simulink library "ddm"  (R2021b)
settings: Solver=VariableStepAuto  StartTime=0.0  StopTime=10.0  RelTol=1e-3
undefined symbols (not defined in the file or in its folder): ENUM_ADASACCSTA_ERROR, ENUM_ADASACCSTA_OFF, ENUM_ADASACCSTA_STANDBY, ENUM_ADASISASTA_OFF, ENUM_ALLOWMOV_ALLOWREADY, ENUM_APS, ENUM_BRKSTA_ERROR, ENUM_BRKSTA_OFF, ENUM_BRKSTA_ON, ENUM_CHGPREACTERRSTA_OBCPRE, ENUM_DCDCFAULTSTA_ANYFAULTLV1, ENUM_DCDCFAULTSTA_ANYFAULTLV2, ENUM_DRIVETRAIN_AWD, ENUM_DRIVETRAIN_FWD, ENUM_DRIVETRAIN_RWD, ENUM_DRSEATSTA_INVALID, ENUM_EDUDRTSTA_NORMAL, ENUM_EPBSTA_APPLIED, ENUM_EPBSTA_RELEASED, ENUM_HVBATTREADYPRE_READY, ENUM_MCUWARN_LV0, ENUM_MCUWARN_LV1, ENUM_MCUWARN_LV2, ENUM_MCUWARN_LV3, ENUM_MCUWARN_NOERROR, ENUM_OBCFAULTSTA_ANYFAULT, ENUM_PAS_R2F2, ENUM_PDFAULT_BATTPDFAIL, ENUM_PDFAULT_DCDCDISABLE, ENUM_PDFAULT_MCUDISABLE, ENUM_PDFAULT_MCUDISCHRG, ENUM_POWERSTA_OFF, ENUM_POWERSTA_ON, ENUM_POWERSTA_READY, ENUM_POWERSTA_STANDBY, ENUM_PRESSINDI_LOW, ENUM_PUFAULT_BATTUPFAIL, ENUM_PUFAULT_DCDCENABLEFAIL, ENUM_PUFAULT_PRECHRGCHKFAIL, ENUM_PUFAULT_SAFETYCHKFAIL, ENUM_PUSTATE_COMPLETED, ENUM_PWRSTASW_OFF, ENUM_PWRSTASW_OFFA, ENUM_PWRSTASW_OFFCHVCHRG, ENUM_PWRSTASW_OFFCLVCHRG, ENUM_PWRSTASW_ON, ENUM_PWRSTASW_ONHVCHRG, ENUM_PWRSTASW_READY, ENUM_PWRSTASW_STANDBY, ENUM_RANGESTA_12IN, ENUM_RANGESTA_12OUT, ENUM_SHIFTCOMMAND_D, ENUM_SHIFTCOMMAND_N, ENUM_SHIFTCOMMAND_P, ENUM_SHIFTCOMMAND_R, ENUM_ZONEMALFUNLV_1ST, ENUM_ZONEMALFUNLV_2ND, ENUM_ZONEMALFUNLV_3RD, ENUM_ZONEMALFUNLV_4TH, ENUM_ZONESPDCTRLMODE_ACC ... (+832)
libraries: hcu_lib x738, $bdroot x26, simulink x7
(part 11 of 25)

== system ddm/DDM/DDM/TQD/Shifter1_DDM ==
  note: Shifter1 Lost Comm (Shifter1NoCom)
  note: Shifter1 Rolling Count Error (Shifter1RCErr)
  note: Shifter1 Rolling Count Error (Shifter1CSErr)
  task_time_s : Inport
  VPMM_SysPwrSta_enum : Inport  Port=2
  No_CAN3_BUS_OFF : Inport  Port=3
  VDDM_Shifter1NoCom_flg : Inport  Port=4
  VDDM_Shifter1RCErr_flg : Inport  Port=5
  VDDM_Shifter1CSErr_flg : Inport  Port=6
  DTC_clear_request : Inport  Port=7
  Constant1 : Constant  Value=KDDM_Shifter1NoComCFSSW_flg
  Constant10 : Constant  Value=KDDM_Shifter1RCErrDFSSW_flg
  Constant{3,11,17,19,31,36} (6 alike) : Constant  Value=ENUM_PWRSTASW_OFF
  Constant12 : Constant  Value=FALSE
  Constant13 : Constant  Value=KDDM_Shifter1RCErrDTC_cnt
  Constant14 : Constant  Value=KDDM_Shifter1RCErrPassTO_s
  Constant15 : Constant  Value=KDDM_Shifter1NoComDTC_cnt
  Constant16 : Constant  Value=KDDM_Shifter1NoComDFSSW_flg
  Constant18 : Constant  Value=KDDM_Shifter1RCErrDetTO_s
  Constant2 : Constant  Value=FALSE
  Constant20 : Constant  Value=KDDM_Shifter1NoComDTC_cnt
  Constant21 : Constant  Value=KDDM_Shifter1NoComPassTO_s
  Constant22 : Constant  Value=KDDM_Shifter1NoComDetTO_s
  Constant23 : Constant  Value=ENUM_POWERSTA_OFF
  Constant24 : Constant  Value=ENUM_POWERSTA_STANDBY
  Constant25 : Constant  Value=KDDM_Shifter1RCErrDetSW_flg
  Constant26 : Constant  Value=KDDM_Shifter1RCErrPassSW_flg
  Constant27 : Constant  Value=KDDM_Shifter1RCErrPassTO_s
  Constant28 : Constant  Value=KDDM_Shifter1CSErrCFSSW_flg
  Constant29 : Constant  Value=KDDM_Shifter1CSErrDTC_cnt
  Constant30 : Constant  Value=KDDM_Shifter1CSErrDFSSW_flg
  Constant32 : Constant  Value=FALSE
  Constant33 : Constant  Value=KDDM_Shifter1CSErrDTC_cnt
  Constant34 : Constant  Value=KDDM_Shifter1CSErrPassTO_s
  Constant35 : Constant  Value=KDDM_Shifter1CSErrDetTO_s
  Constant37 : Constant  Value=ENUM_POWERSTA_OFF
  Constant38 : Constant  Value=ENUM_POWERSTA_STANDBY
  Constant39 : Constant  Value=KDDM_Shifter1CSErrDetSW_flg
  Constant4 : Constant  Value=ENUM_POWERSTA_OFF
  Constant40 : Constant  Value=KDDM_Shifter1CSErrPassSW_flg
  Constant41 : Constant  Value=KDDM_Shifter1CSErrPassTO_s
  Constant5 : Constant  Value=ENUM_POWERSTA_STANDBY
  Constant6 : Constant  Value=KDDM_Shifter1NoComDetSW_flg
  Constant7 : Constant  Value=KDDM_Shifter1NoComPassSW_flg
  Constant70 : Constant  Value=KDDM_Shifter1NoComPassTO_s
  Constant8 : Constant  Value=KDDM_Shifter1RCErrCFSSW_flg
  Constant9 : Constant  Value=KDDM_Shifter1RCErrDTC_cnt
  DTC_Couter1 : hcu_lib/Basic_Blocks/DTC_Couter
  DTC_Couter2 : hcu_lib/Basic_Blocks/DTC_Couter
  DTC_Couter3 : hcu_lib/Basic_Blocks/DTC_Couter
  DTC_Info : hcu_lib/Basic_Blocks/DTC_Info
  DTC_Info1 : hcu_lib/Basic_Blocks/DTC_Info
  DTC_Info2 : hcu_lib/Basic_Blocks/DTC_Info
  Data Type Conversion1 : DataTypeConversion  OutDataTypeStr=uint8
  Data Type Conversion2 : DataTypeConversion  OutDataTypeStr=uint8
  Data Type Conversion3 : DataTypeConversion  OutDataTypeStr=uint8
  Equal{1,3,9..12} (6 alike) : RelationalOperator  Operator===  OutDataTypeStr=boolean  RndMeth=Simplest
  Equal{2,4..6,13..14} (6 alike) : RelationalOperator  Operator=~=  OutDataTypeStr=boolean  RndMeth=Simplest
  Equal15 : RelationalOperator  OutDataTypeStr=boolean  RndMeth=Simplest
  Equal7 : RelationalOperator  OutDataTypeStr=boolean  RndMeth=Simplest
  Equal8 : RelationalOperator  OutDataTypeStr=boolean  RndMeth=Simplest
  Logical Operator{1,3,5,11,23,25,27,37,77} (9 alike) : Logic  Operator=OR  AllPortsSameDT=off  OutDataTypeStr=boolean
  Logical Operator10 : Logic  Inputs=3  AllPortsSameDT=off  OutDataTypeStr=boolean
  Logical Operator{6,9,12,14,20,24,28,30,34,38} (10 alike) : Logic  Operator=NOT  AllPortsSameDT=off  OutDataTypeStr=boolean
  Logical Operator{2,8,13,15..19,21,29,31..33,35,55} (15 alike) : Logic  AllPortsSameDT=off  OutDataTypeStr=boolean
  Logical Operator{4,22,26,36} (4 alike) : Logic  Inputs=4  AllPortsSameDT=off  OutDataTypeStr=boolean
  Logical Operator7 : Logic  Inputs=3  AllPortsSameDT=off  OutDataTypeStr=boolean
  Relay1 : Relay  OnSwitchValue=ONE_INT  OffSwitchValue=ZERO_INT
  Relay2 : Relay  OnSwitchValue=ONE_INT  OffSwitchValue=ZERO_INT
  Relay3 : Relay  OnSwitchValue=ONE_INT  OffSwitchValue=ZERO_INT
  SR_Latch{1..8,12} (9 alike) : hcu_lib/Basic_Blocks/SR_Latch
  Switch1 : Switch  Criteria=u2 ~= 0
  Switch2 : Switch  Criteria=u2 ~= 0
  Switch6 : Switch  Criteria=u2 ~= 0
  Test Detection Criteria1 : hcu_lib/Basic_Blocks/Test Detection Criteria
  Test Detection Criteria2 : hcu_lib/Basic_Blocks/Test Detection Criteria
  Test Detection Criteria3 : hcu_lib/Basic_Blocks/Test Detection Criteria
  Timer1 : hcu_lib/Basic_Blocks/Timer
  Timer2 : hcu_lib/Basic_Blocks/Timer
  Timer3 : hcu_lib/Basic_Blocks/Timer
  Unit Delay1 : UnitDelay  SampleTime=-1  HasFrameUpgradeWarning=on
  Unit Delay2 : UnitDelay  SampleTime=-1  HasFrameUpgradeWarning=on
  Unit Delay3 : UnitDelay  SampleTime=-1  HasFrameUpgradeWarning=on
  VDDM_Shifter1NoComDTC_raw32 : Outport
  VDDM_Shifter1RCErrDTC_raw32 : Outport  Port=2
  VDDM_Shifter1CSErrDTC_raw32 : Outport  Port=3
  wires:
  Logical Operator77/1 -> SR_Latch2/2
  [DTC_clear_request] -> Logical Operator1/2
  SR_Latch2/1 -> Logical Operator55/2
  Logical Operator14/1 -> Timer2/2
  [VDDM_Shifter1NoComCFSRls_flg] -> SR_Latch1/2
  Logical Operator13/1 -> Logical Operator1/1
  Relay1/1 -> SR_Latch2/1
  Constant22/1 -> Test Detection Criteria1/4
  Logical Operator16/1 -> DTC_Couter1/2
  Logical Operator7/1 -> Logical Operator14/1, Timer2/1
  Timer2/1 -> Equal7/1
  Equal10/1 -> Logical Operator13/1
  SR_Latch12/1 -> [VDDM_Shifter1NoComPass_flg]
  DTC_Couter1/2 -> Data Type Conversion2/1
  Constant4/1 -> Equal10/2
  [VDDM_Shifter1NoComDet_flg] -> Logical Operator15/1
  Constant6/1 -> Logical Operator15/2
  Test Detection Criteria1/1 -> [VDDM_Shifter1NoComDet_flg]  "VDDM_Shifter1NoComDet_flg"
  Logical Operator15/1 -> DTC_Couter1/1
  [VDDM_Shifter1NoComCFSRls_flg] -> Logical Operator11/2
  [VDDM_Shifter1NoComDFSRls_flg] -> Logical Operator77/1
  [VDDM_Shifter1NoComPass_flg] -> Logical Operator11/1
  [VDDM_Shifter1NoComDTC_cnt] -> Relay1/1
  Constant20/1 -> Test Detection Criteria1/3
  [VDDM_Shifter1NoComCFS_flg] -> Logical Operator77/2
  [VPMM_SysPwrSta_enum] -> Equal11/1
  Equal7/1 -> SR_Latch12/1
  Equal11/1 -> Logical Operator13/2
  Unit Delay2/1 -> Equal10/1
  Logical Operator11/1 -> Logical Operator16/1
  Constant16/1 -> Logical Operator55/1
  Data Type Conversion2/1 -> [VDDM_Shifter1NoComDTC_cnt]  "VDDM_Shifter1NoComDTC_cnt"
  Logical Operator55/1 -> [VDDM_Shifter1NoComDFS_flg]
  Constant15/1 -> DTC_Couter1/3
  Constant5/1 -> Equal11/2
  Constant7/1 -> Logical Operator16/2
  Logical Operator1/1 -> [VDDM_Shifter1NoComCFSRls_flg]
  Constant70/1 -> Timer2/4
  DTC_Couter1/1 -> SR_Latch1/1
  [VPMM_SysPwrSta_enum] -> Unit Delay2/1
  [task_time_s] -> Test Detection Criteria1/2
  Constant21/1 -> Equal7/2
  [task_time_s] -> Timer2/3
  [No_CAN3_BUS_OFF] -> Logical Operator10/2
  Equal6/1 -> Logical Operator10/1
  Constant17/1 -> Equal6/2
  [VDDM_Shifter1NoCom_flg] -> Logical Operator10/3
  [VPMM_SysPwrSta_enum] -> Equal6/1
  [VDDM_Shifter1NoCom_flg] -> Logical Operator9/1
  Equal2/1 -> Logical Operator7/1
  Logical Operator9/1 -> Logical Operator7/3
  Constant3/1 -> Equal2/2
  [No_CAN3_BUS_OFF] -> Logical Operator7/2
  [VPMM_SysPwrSta_enum] -> Equal2/1
  VDDM_Shifter1NoCom_flg/1 -> [VDDM_Shifter1NoCom_flg]
  VPMM_SysPwrSta_enum/1 -> [VPMM_SysPwrSta_enum]
  [VDDM_Shifter1NoComCFS_flg] -> DTC_Info/3
  DTC_Info/1 -> VDDM_Shifter1NoComDTC_raw32/1  "VDDM_Shifter1NoComDTC_raw32"
  [VDDM_Shifter1NoComPass_flg] -> DTC_Info/2
  task_time_s/1 -> [task_time_s]
  DTC_clear_request/1 -> [DTC_clear_request]
  [VDDM_Shifter1NoComDet_flg] -> DTC_Info/1
  No_CAN3_BUS_OFF/1 -> [No_CAN3_BUS_OFF]
  Constant1/1 -> Logical Operator2/2
  Logical Operator2/1 -> [VDDM_Shifter1NoComCFS_flg]
  SR_Latch1/1 -> Logical Operator2/1
  [DTC_clear_request] -> DTC_Info/4
  [DTC_clear_request] -> Switch6/2
  Switch6/1 -> Test Detection Criteria1/1
  Logical Operator10/1 -> [VDDM_Shifter1NoComRst_flg], Switch6/3
  Constant2/1 -> Switch6/1
  Logical Operator20/1 -> Logical Operator4/4
  [DTC_clear_request] -> Logical Operator3/2
  Constant26/1 -> Logical Operator18/2
  Logical Operator12/1 -> Timer1/2
  SR_Latch5/1 -> Logical Operator21/2
  [VPMM_SysPwrSta_enum] -> Equal4/1
  [VDDM_Shifter1RCErrPass_flg] -> Logical Operator5/1
  Logical Operator8/1 -> Logical Operator3/1
  Logical Operator19/1 -> [VDDM_Shifter1RCErrCFS_flg]
  Constant13/1 -> Test Detection Criteria2/3
  Equal1/1 -> Logical Operator8/1
  Constant25/1 -> Logical Operator17/2
  Logical Operator5/1 -> Logical Operator18/1
  SR_Latch4/1 -> [VDDM_Shifter1RCErrPass_flg]
  Logical Operator17/1 -> DTC_Couter2/1
  [VDDM_Shifter1RCErrCFS_flg] -> Logical Operator23/2
  DTC_Couter2/2 -> Data Type Conversion1/1
  Equal5/1 -> Logical Operator4/1
  Logical Operator22/1 -> Timer1/1, Logical Operator12/1
  Unit Delay1/1 -> Equal1/1
  [VDDM_Shifter1NoComCFS_flg] -> Logical Operator20/1
  Constant24/1 -> Equal3/2
  Logical Operator21/1 -> [VDDM_Shifter1RCErrDFS_flg]
  Constant14/1 -> Equal8/2
  [VDDM_Shifter1RCErr_flg] -> Logical Operator24/1
  Logical Operator3/1 -> [VDDM_Shifter1RCErrCFSRls_flg]
  Constant19/1 -> Equal4/2
  Equal8/1 -> SR_Latch4/1
  [VDDM_Shifter1RCErrCFSRls_flg] -> SR_Latch3/2
  Constant11/1 -> Equal5/2
  Constant18/1 -> Test Detection Criteria2/4
  [VDDM_Shifter1RCErrPass_flg] -> DTC_Info1/2
  [No_CAN3_BUS_OFF] -> Logical Operator22/2
  Equal4/1 -> Logical Operator22/1
  Constant23/1 -> Equal1/2
  Logical Operator18/1 -> DTC_Couter2/2
  Data Type Conversion1/1 -> [VDDM_Shifter1RCErrDTC_cnt]  "VDDM_Shifter1RCErrDTC_cnt"
  DTC_Info1/1 -> VDDM_Shifter1RCErrDTC_raw32/1  "VDDM_Shifter1RCErrDTC_raw32"
  Constant10/1 -> Logical Operator21/1
  Logical Operator23/1 -> SR_Latch5/2
  [VPMM_SysPwrSta_enum] -> Equal3/1
  [VPMM_SysPwrSta_enum] -> Equal5/1
  [No_CAN3_BUS_OFF] -> Logical Operator4/2
  [VDDM_Shifter1RCErrDet_flg] -> DTC_Info1/1
  Relay2/1 -> SR_Latch5/1
  [VDDM_Shifter1RCErrDet_flg] -> Logical Operator17/1
  [task_time_s] -> Timer1/3
  [task_time_s] -> Test Detection Criteria2/2
  Constant27/1 -> Timer1/4
  Timer1/1 -> Equal8/1
  SR_Latch3/1 -> Logical Operator19/1
  [DTC_clear_request] -> Switch1/2
  Constant12/1 -> Switch1/1
  Equal3/1 -> Logical Operator8/2
  [VDDM_Shifter1RCErrDTC_cnt] -> Relay2/1
  [VDDM_Shifter1RCErrCFS_flg] -> DTC_Info1/3
  [VPMM_SysPwrSta_enum] -> Unit Delay1/1
  Constant9/1 -> DTC_Couter2/3
  Logical Operator4/1 -> [VDDM_Shifter1RCErrRst_flg], Switch1/3
  [VDDM_Shifter1RCErrDFSRls_flg] -> Logical Operator23/1
  [VDDM_Shifter1RCErrCFSRls_flg] -> Logical Operator5/2
  Logical Operator24/1 -> Logical Operator22/3
  DTC_Couter2/1 -> SR_Latch3/1
  [DTC_clear_request] -> DTC_Info1/4
  Constant8/1 -> Logical Operator19/2
  [VDDM_Shifter1RCErr_flg] -> Logical Operator4/3
  Test Detection Criteria2/1 -> [VDDM_Shifter1RCErrDet_flg]  "VDDM_Shifter1RCErrDet_flg"
  Logical Operator34/1 -> Logical Operator26/4
  [DTC_clear_request] -> Logical Operator25/2
  Constant40/1 -> Logical Operator32/2
  Logical Operator30/1 -> Timer3/2
  SR_Latch8/1 -> Logical Operator35/2
  [VPMM_SysPwrSta_enum] -> Equal13/1
  [VDDM_Shifter1CSErrPass_flg] -> Logical Operator27/1
  Logical Operator29/1 -> Logical Operator25/1
  Logical Operator33/1 -> [VDDM_Shifter1CSErrCFS_flg]
  Constant33/1 -> Test Detection Criteria3/3
  Equal9/1 -> Logical Operator29/1
  Constant39/1 -> Logical Operator31/2
  Logical Operator27/1 -> Logical Operator32/1
  SR_Latch7/1 -> [VDDM_Shifter1CSErrPass_flg]
  Logical Operator31/1 -> DTC_Couter3/1
  [VDDM_Shifter1CSErrCFS_flg] -> Logical Operator37/2
  DTC_Couter3/2 -> Data Type Conversion3/1
  Equal14/1 -> Logical Operator26/1
  Logical Operator36/1 -> Timer3/1, Logical Operator30/1
  Unit Delay3/1 -> Equal9/1
  [VDDM_Shifter1NoComCFS_flg] -> Logical Operator34/1
  Constant38/1 -> Equal12/2
  Logical Operator35/1 -> [VDDM_Shifter1CSErrDFS_flg]
  Constant34/1 -> Equal15/2
  [VDDM_Shifter1CSErr_flg] -> Logical Operator38/1
  Logical Operator25/1 -> [VDDM_Shifter1CSErrCFSRls_flg]
  Constant36/1 -> Equal13/2
  Equal15/1 -> SR_Latch7/1
  [VDDM_Shifter1CSErrCFSRls_flg] -> SR_Latch6/2
  Constant31/1 -> Equal14/2
  Constant35/1 -> Test Detection Criteria3/4
  [VDDM_Shifter1CSErrPass_flg] -> DTC_Info2/2
  [No_CAN3_BUS_OFF] -> Logical Operator36/2
  Equal13/1 -> Logical Operator36/1
  Constant37/1 -> Equal9/2
  Logical Operator32/1 -> DTC_Couter3/2
  Data Type Conversion3/1 -> [VDDM_Shifter1CSErrDTC_cnt]  "VDDM_Shifter1CSErrDTC_cnt"
  DTC_Info2/1 -> VDDM_Shifter1CSErrDTC_raw32/1  "VDDM_Shifter1CSErrDTC_raw32"
  Constant30/1 -> Logical Operator35/1
  Logical Operator37/1 -> SR_Latch8/2
  [VPMM_SysPwrSta_enum] -> Equal12/1
  [VPMM_SysPwrSta_enum] -> Equal14/1
  [No_CAN3_BUS_OFF] -> Logical Operator26/2
  [VDDM_Shifter1CSErrDet_flg] -> DTC_Info2/1
  Relay3/1 -> SR_Latch8/1
  [VDDM_Shifter1CSErrDet_flg] -> Logical Operator31/1
  [task_time_s] -> Timer3/3
  [task_time_s] -> Test Detection Criteria3/2
  Constant41/1 -> Timer3/4
  Timer3/1 -> Equal15/1
  SR_Latch6/1 -> Logical Operator33/1
  [DTC_clear_request] -> Switch2/2
  Constant32/1 -> Switch2/1
  Equal12/1 -> Logical Operator29/2
  [VDDM_Shifter1CSErrDTC_cnt] -> Relay3/1
  [VDDM_Shifter1CSErrCFS_flg] -> DTC_Info2/3
  [VPMM_SysPwrSta_enum] -> Unit Delay3/1
  Constant29/1 -> DTC_Couter3/3
  Logical Operator26/1 -> [VDDM_Shifter1CSErrRst_flg], Switch2/3
  [VDDM_Shifter1CSErrDFSRls_flg] -> Logical Operator37/1
  [VDDM_Shifter1CSErrCFSRls_flg] -> Logical Operator27/2
  Logical Operator38/1 -> Logical Operator36/3
  DTC_Couter3/1 -> SR_Latch6/1
  [DTC_clear_request] -> DTC_Info2/4
  Constant28/1 -> Logical Operator33/2
  [VDDM_Shifter1CSErr_flg] -> Logical Operator26/3
  Test Detection Criteria3/1 -> [VDDM_Shifter1CSErrDet_flg]  "VDDM_Shifter1CSErrDet_flg"
  [VDDM_Shifter1NoComRst_flg] -> SR_Latch12/2
  Switch1/1 -> Test Detection Criteria2/1
  [VDDM_Shifter1RCErrRst_flg] -> SR_Latch4/2
  [VDDM_Shifter1CSErrRst_flg] -> SR_Latch7/2
  Switch2/1 -> Test Detection Criteria3/1
  VDDM_Shifter1RCErr_flg/1 -> [VDDM_Shifter1RCErr_flg]
  VDDM_Shifter1CSErr_flg/1 -> [VDDM_Shifter1CSErr_flg]
  [VDDM_Shifter1NoComCFS_flg] -> Logical Operator6/1
  Logical Operator6/1 -> Logical Operator22/4
  [VDDM_Shifter1NoComCFS_flg] -> Logical Operator28/1
  Logical Operator28/1 -> Logical Operator36/4

== system ddm/DDM/DDM/VMC_DDM/ACC Acceleration Command Error ==
  task_time_s : Inport
  VDDM_FCM2NoComCFS_flg : Inport  Port=2
  VDDM_FCM2RCErrCFS_flg : Inport  Port=3
  VDDM_FCM2CSErrCFS_flg : Inport  Port=4
  VVMC_ADASActive_flg : Inport  Port=5
  No_CAN_BUS_OFF : Inport  Port=6
  VPMM_PowerSta_enum : Inport  Port=7
  VINP_ACCRequireAccel_mps2 : Inport  Port=8
  VINP_ADASACCSta_enum : Inport  Port=9
  DTC_clear_request : Inport  Port=10
  "ACC Acceleration Command Error " : Subsystem
  From5 : From  Commented=on  GotoTag=VDDM_ACCAccelCmdErrDFS_flg
  Terminator : Terminator
  VDDM_ACCAccelCmdErrCFS_flg : Outport
  VDDM_ACCAccelCmdErrDetDTC_raw32 : Outport  Port=2
  wires:
  VDDM_FCM2CSErrCFS_flg/1 -> [VDDM_FCM2CSErrCFS_flg]
  VDDM_FCM2RCErrCFS_flg/1 -> [VDDM_FCM2RCErrCFS_flg]
  [VDDM_ACCAccelCmdErrCFS_flg] -> VDDM_ACCAccelCmdErrCFS_flg/1
  From5/1 -> Terminator/1
  "ACC Acceleration Command Error "/1(VDDM_ACCAccelCmdErrCFS_flg) -> [VDDM_ACCAccelCmdErrCFS_flg]
  DTC_clear_request/1 -> [DTC_clear_request]
  VPMM_PowerSta_enum/1 -> [VPMM_PowerSta_enum]
  No_CAN_BUS_OFF/1 -> [No_CAN_BUS_OFF]
  VDDM_FCM2NoComCFS_flg/1 -> [VDDM_FCM2NoComCFS_flg]
  VINP_ACCRequireAccel_mps2/1 -> [VINP_ACCRequireAccel_mps2]
  [VDDM_FCM2NoComCFS_flg] -> "ACC Acceleration Command Error "/2(VDDM_FCM2NoComCFS_flg)
  [VDDM_FCM2RCErrCFS_flg] -> "ACC Acceleration Command Error "/3(VDDM_FCM2RCErrCFS_flg)
  [VDDM_FCM2CSErrCFS_flg] -> "ACC Acceleration Command Error "/4(VDDM_FCM2CSErrCFS_flg)
  [No_CAN_BUS_OFF] -> "ACC Acceleration Command Error "/6(No_CAN_BUS_OFF)
  [VPMM_PowerSta_enum] -> "ACC Acceleration Command Error "/7(VPMM_PowerSta_enum)
  [VINP_ACCRequireAccel_mps2] -> "ACC Acceleration Command Error "/8(VINP_ACCRequireAccel_mps2)
  [DTC_clear_request] -> "ACC Acceleration Command Error "/10(DTC_clear_request)
  task_time_s/1 -> [task_time_s]  "task_time_s"
  [task_time_s] -> "ACC Acceleration Command Error "/1(task_time_s)
  VVMC_ADASActive_flg/1 -> [VVMC_ADASActive_flg]
  [VVMC_ADASActive_flg] -> "ACC Acceleration Command Error "/5(VVMC_ADASActive_flg)
  [VINP_ADASACCSta_enum] -> "ACC Acceleration Command Error "/9(VINP_ADASACCSta_enum)
  VINP_ADASACCSta_enum/1 -> [VINP_ADASACCSta_enum]
  "ACC Acceleration Command Error "/2(VDDM_ACCAccelCmdErrDetDTC_raw32) -> [VDDM_ACCAccelCmdErrDetDTC_raw32]
  [VDDM_ACCAccelCmdErrDetDTC_raw32] -> VDDM_ACCAccelCmdErrDetDTC_raw32/1

== system ddm/DDM/DDM/VMC_DDM/ACC Malfunction  ==
  task_time_s : Inport
  VDDM_FCMACCSigErrCFS_flg : Inport  Port=2
  VDDM_ACCAccelCmdErrCFS_flg : Inport  Port=3
  VDDM_BMSSigErrCFS_flg : Inport  Port=4
  VDDM_FrMCUSigErrCFS_flg : Inport  Port=5
  VDDM_RrMCUSigErrCFS_flg : Inport  Port=6
  VDDM_CCUSigErrCFS_flg : Inport  Port=7
  VDDM_FCM2NoComCFS_flg : Inport  Port=8
  VDDM_FCM2RCErrCFS_flg : Inport  Port=9
  VDDM_FCM2CSErrCFS_flg : Inport  Port=10
  VDDM_FCM4NoComCFS_flg : Inport  Port=11
  VDDM_FCM4CSErrCFS_flg : Inport  Port=12
  VDDM_ZoneSCPNoComCFS_flg : Inport  Port=13
  VDDM_MCUR1NoComCFS_flg : Inport  Port=14
  VDDM_MCUR1RCErrCFS_flg : Inport  Port=15
  VDDM_MCUR1CSErrCFS_flg : Inport  Port=16
  VDDM_MCUF1NoComCFS_flg : Inport  Port=17
  VDDM_MCUF1RCErrCFS_flg : Inport  Port=18
  VDDM_MCUF1CSErrCFS_flg : Inport  Port=19
  VDDM_ESC7NoComCFS_flg : Inport  Port=20
  VDDM_ESC7RCErrCFS_flg : Inport  Port=21
  VDDM_ESC7CSErrCFS_flg : Inport  Port=22
  VDDM_ESC1NoComCFS_flg : Inport  Port=23
  VDDM_ESC1RCErrCFS_flg : Inport  Port=24
  VDDM_ESC1CSErrCFS_flg : Inport  Port=25
  VDDM_ESC5NoComCFS_flg : Inport  Port=26
  VDDM_ESC5RCErrCFS_flg : Inport  Port=27
  VDDM_ESC5CSErrCFS_flg : Inport  Port=28
  No_CAN1_BUS_OFF : Inport  Port=29
  No_CAN3_BUS_OFF : Inport  Port=30
  No_CAN4_BUS_OFF : Inport  Port=31
  VPMM_PowerSta_enum : Inport  Port=32
  VINP_ZoneSpdCtrlMode_enum : Inport  Port=33
  DTC_clear_request : Inport  Port=34
  "ACC Malfunction " : Subsystem
  From5 : From  Commented=on  GotoTag=VDDM_ACCMalfuncDFS_flg
  Terminator : Terminator
  VDDM_ACCMalfuncCFS_flg : Outport
  VDDM_ACCMalfuncDetDTC_raw32 : Outport  Port=2
  wires:
  VDDM_BMSSigErrCFS_flg/1 -> [VDDM_BMSSigErrCFS_flg]
  VDDM_ACCAccelCmdErrCFS_flg/1 -> [VDDM_ACCAccelCmdErrCFS_flg]
  [VDDM_ACCMalfuncCFS_flg] -> VDDM_ACCMalfuncCFS_flg/1
  From5/1 -> Terminator/1
  "ACC Malfunction "/1(VDDM_ACCMalfuncCFS_flg) -> [VDDM_ACCMalfuncCFS_flg]
  VPMM_PowerSta_enum/1 -> [VPMM_PowerSta_enum]
  No_CAN1_BUS_OFF/1 -> [No_CAN1_BUS_OFF]
  VDDM_FCMACCSigErrCFS_flg/1 -> [VDDM_FCMACCSigErrCFS_flg]
  VINP_ZoneSpdCtrlMode_enum/1 -> [VINP_ZoneSpdCtrlMode_enum]
  task_time_s/1 -> [task_time_s]  "task_time_s"
  VDDM_FrMCUSigErrCFS_flg/1 -> [VDDM_FrMCUSigErrCFS_flg]
  VDDM_RrMCUSigErrCFS_flg/1 -> [VDDM_RrMCUSigErrCFS_flg]
  VDDM_CCUSigErrCFS_flg/1 -> [VDDM_CCUSigErrCFS_flg]
  VDDM_ZoneSCPNoComCFS_flg/1 -> [VDDM_ZoneSCPNoComCFS_flg]
  VDDM_FCM4CSErrCFS_flg/1 -> [VDDM_FCM4CSErrCFS_flg]
  VDDM_FCM4NoComCFS_flg/1 -> [VDDM_FCM4NoComCFS_flg]
  VDDM_FCM2NoComCFS_flg/1 -> [VDDM_FCM2NoComCFS_flg]
  VDDM_FCM2RCErrCFS_flg/1 -> [VDDM_FCM2RCErrCFS_flg]
  VDDM_FCM2CSErrCFS_flg/1 -> [VDDM_FCM2CSErrCFS_flg]
  VDDM_ESC7CSErrCFS_flg/1 -> [VDDM_ESC7CSErrCFS_flg]
  VDDM_ESC7RCErrCFS_flg/1 -> [VDDM_ESC7RCErrCFS_flg]
  VDDM_ESC7NoComCFS_flg/1 -> [VDDM_ESC7NoComCFS_flg]
  VDDM_ESC1NoComCFS_flg/1 -> [VDDM_ESC1NoComCFS_flg]
  VDDM_ESC1RCErrCFS_flg/1 -> [VDDM_ESC1RCErrCFS_flg]
  VDDM_ESC1CSErrCFS_flg/1 -> [VDDM_ESC1CSErrCFS_flg]
  VDDM_MCUF1CSErrCFS_flg/1 -> [VDDM_MCUF1CSErrCFS_flg]
  VDDM_MCUF1RCErrCFS_flg/1 -> [VDDM_MCUF1RCErrCFS_flg]
  VDDM_MCUF1NoComCFS_flg/1 -> [VDDM_MCUF1NoComCFS_flg]
  VDDM_MCUR1NoComCFS_flg/1 -> [VDDM_MCUR1NoComCFS_flg]
  VDDM_MCUR1RCErrCFS_flg/1 -> [VDDM_MCUR1RCErrCFS_flg]
  VDDM_MCUR1CSErrCFS_flg/1 -> [VDDM_MCUR1CSErrCFS_flg]
  VDDM_ESC5CSErrCFS_flg/1 -> [VDDM_ESC5CSErrCFS_flg]
  VDDM_ESC5RCErrCFS_flg/1 -> [VDDM_ESC5RCErrCFS_flg]
  VDDM_ESC5NoComCFS_flg/1 -> [VDDM_ESC5NoComCFS_flg]
  No_CAN3_BUS_OFF/1 -> [No_CAN3_BUS_OFF]
  No_CAN4_BUS_OFF/1 -> [No_CAN4_BUS_OFF]
  DTC_clear_request/1 -> [DTC_clear_request]
  [No_CAN3_BUS_OFF] -> "ACC Malfunction "/30(No_CAN3_BUS_OFF)
  [VDDM_MCUR1CSErrCFS_flg] -> "ACC Malfunction "/16(VDDM_MCUR1CSErrCFS_flg)
  [VDDM_RrMCUSigErrCFS_flg] -> "ACC Malfunction "/6(VDDM_RrMCUSigErrCFS_flg)
  [VDDM_BMSSigErrCFS_flg] -> "ACC Malfunction "/4(VDDM_BMSSigErrCFS_flg)
  [VDDM_MCUF1NoComCFS_flg] -> "ACC Malfunction "/17(VDDM_MCUF1NoComCFS_flg)
  [No_CAN4_BUS_OFF] -> "ACC Malfunction "/31(No_CAN4_BUS_OFF)
  [VDDM_FrMCUSigErrCFS_flg] -> "ACC Malfunction "/5(VDDM_FrMCUSigErrCFS_flg)
  [DTC_clear_request] -> "ACC Malfunction "/34(DTC_clear_request)
  [VDDM_ACCAccelCmdErrCFS_flg] -> "ACC Malfunction "/3(VDDM_ACCAccelCmdErrCFS_flg)
  [VDDM_MCUF1RCErrCFS_flg] -> "ACC Malfunction "/18(VDDM_MCUF1RCErrCFS_flg)
  [VDDM_ESC7CSErrCFS_flg] -> "ACC Malfunction "/22(VDDM_ESC7CSErrCFS_flg)
  [VDDM_FCM4CSErrCFS_flg] -> "ACC Malfunction "/12(VDDM_FCM4CSErrCFS_flg)
  [VDDM_ESC1RCErrCFS_flg] -> "ACC Malfunction "/24(VDDM_ESC1RCErrCFS_flg)
  [VDDM_ESC7RCErrCFS_flg] -> "ACC Malfunction "/21(VDDM_ESC7RCErrCFS_flg)
  [VDDM_ESC7NoComCFS_flg] -> "ACC Malfunction "/20(VDDM_ESC7NoComCFS_flg)
  [VDDM_ESC5CSErrCFS_flg] -> "ACC Malfunction "/28(VDDM_ESC5CSErrCFS_flg)
  [VDDM_ESC5RCErrCFS_flg] -> "ACC Malfunction "/27(VDDM_ESC5RCErrCFS_flg)
  [VDDM_ESC1NoComCFS_flg] -> "ACC Malfunction "/23(VDDM_ESC1NoComCFS_flg)
  [VDDM_ESC1CSErrCFS_flg] -> "ACC Malfunction "/25(VDDM_ESC1CSErrCFS_flg)
  [No_CAN1_BUS_OFF] -> "ACC Malfunction "/29(No_CAN1_BUS_OFF)
  [VDDM_FCMACCSigErrCFS_flg] -> "ACC Malfunction "/2(VDDM_FCMACCSigErrCFS_flg)
  [VPMM_PowerSta_enum] -> "ACC Malfunction "/32(VPMM_PowerSta_enum)
  [task_time_s] -> "ACC Malfunction "/1(task_time_s)
  [VDDM_MCUF1CSErrCFS_flg] -> "ACC Malfunction "/19(VDDM_MCUF1CSErrCFS_flg)
  [VDDM_MCUR1NoComCFS_flg] -> "ACC Malfunction "/14(VDDM_MCUR1NoComCFS_flg)
  [VDDM_FCM2CSErrCFS_flg] -> "ACC Malfunction "/10(VDDM_FCM2CSErrCFS_flg)
  [VDDM_CCUSigErrCFS_flg] -> "ACC Malfunction "/7(VDDM_CCUSigErrCFS_flg)
  [VDDM_FCM2NoComCFS_flg] -> "ACC Malfunction "/8(VDDM_FCM2NoComCFS_flg)
  [VDDM_FCM2RCErrCFS_flg] -> "ACC Malfunction "/9(VDDM_FCM2RCErrCFS_flg)
  [VDDM_ESC5NoComCFS_flg] -> "ACC Malfunction "/26(VDDM_ESC5NoComCFS_flg)
  [VDDM_FCM4NoComCFS_flg] -> "ACC Malfunction "/11(VDDM_FCM4NoComCFS_flg)
  [VINP_ZoneSpdCtrlMode_enum] -> "ACC Malfunction "/33(VINP_ZoneSpdCtrlMode_enum)
  [VDDM_MCUR1RCErrCFS_flg] -> "ACC Malfunction "/15(VDDM_MCUR1RCErrCFS_flg)
  [VDDM_ZoneSCPNoComCFS_flg] -> "ACC Malfunction "/13(VDDM_ZoneSCPNoComCFS_flg)
  "ACC Malfunction "/2(VDDM_ACCMalfuncDetDTC_raw32) -> [VDDM_ACCMalfuncDetDTC_raw32]
  [VDDM_ACCMalfuncDetDTC_raw32] -> VDDM_ACCMalfuncDetDTC_raw32/1

== system ddm/DDM/DDM/VMC_DDM/BMS Signal Error  ==
  task_time_s : Inport
  VDDM_C3BMS6LCCFS_flg : Inport  Port=2
  VDDM_C3BMS6RCCFS_flg : Inport  Port=3
  VDDM_C3BMS6CSCFS_flg : Inport  Port=4
  No_CAN_BUS_OFF : Inport  Port=5
  VPMM_PowerSta_enum : Inport  Port=6
  VINP_BMSWarn8_flg : Inport  Port=7
  VINP_BMSWarn7_flg : Inport  Port=8
  VINP_BMSWarn6_flg : Inport  Port=9
  VINP_BMSWarn5_flg : Inport  Port=10
  VINP_BMSWarn4_flg : Inport  Port=11
  DTC_clear_request : Inport  Port=12
  "BMS Signal Error " : Subsystem
  From5 : From  Commented=on  GotoTag=VDDM_BMSSigErrDFS_flg
  Terminator : Terminator
  VDDM_BMSSigErrCFS_flg : Outport
  VDDM_BMSSigErrDetDTC_raw32 : Outport  Port=2
  wires:
  VDDM_C3BMS6CSCFS_flg/1 -> [VDDM_C3BMS6CSCFS_flg]
  VDDM_C3BMS6RCCFS_flg/1 -> [VDDM_C3BMS6RCCFS_flg]
  [VDDM_BMSSigErrCFS_flg] -> VDDM_BMSSigErrCFS_flg/1
  From5/1 -> Terminator/1
  "BMS Signal Error "/1(VDDM_BMSSigErrCFS_flg) -> [VDDM_BMSSigErrCFS_flg]
  DTC_clear_request/1 -> [DTC_clear_request]
  VPMM_PowerSta_enum/1 -> [VPMM_PowerSta_enum]
  No_CAN_BUS_OFF/1 -> [No_CAN_BUS_OFF]
  VDDM_C3BMS6LCCFS_flg/1 -> [VDDM_C3BMS6LCCFS_flg]
  VINP_BMSWarn8_flg/1 -> [VINP_BMSWarn8_flg]
  VINP_BMSWarn7_flg/1 -> [VINP_BMSWarn7_flg]
  VINP_BMSWarn5_flg/1 -> [VINP_BMSWarn5_flg]
  VINP_BMSWarn6_flg/1 -> [VINP_BMSWarn6_flg]
  VINP_BMSWarn4_flg/1 -> [VINP_BMSWarn4_flg]
  [VDDM_C3BMS6LCCFS_flg] -> "BMS Signal Error "/2(VDDM_C3BMS6LCCFS_flg)
  [VDDM_C3BMS6RCCFS_flg] -> "BMS Signal Error "/3(VDDM_C3BMS6RCCFS_flg)
  [VDDM_C3BMS6CSCFS_flg] -> "BMS Signal Error "/4(VDDM_C3BMS6CSCFS_flg)
  [No_CAN_BUS_OFF] -> "BMS Signal Error "/5(No_CAN_BUS_OFF)
  [VPMM_PowerSta_enum] -> "BMS Signal Error "/6(VPMM_PowerSta_enum)
  [VINP_BMSWarn8_flg] -> "BMS Signal Error "/7(VINP_BMSWarn8_flg)
  [VINP_BMSWarn7_flg] -> "BMS Signal Error "/8(VINP_BMSWarn7_flg)
  [VINP_BMSWarn6_flg] -> "BMS Signal Error "/9(VINP_BMSWarn6_flg)
  [VINP_BMSWarn5_flg] -> "BMS Signal Error "/10(VINP_BMSWarn5_flg)
  [VINP_BMSWarn4_flg] -> "BMS Signal Error "/11(VINP_BMSWarn4_flg)
  [DTC_clear_request] -> "BMS Signal Error "/12(DTC_clear_request)
  task_time_s/1 -> [task_time_s]  "task_time_s"
  [task_time_s] -> "BMS Signal Error "/1(task_time_s)
  "BMS Signal Error "/2(VDDM_BMSSigErrDetDTC_raw32) -> [VDDM_BMSSigErrDetDTC_raw32]
  [VDDM_BMSSigErrDetDTC_raw32] -> VDDM_BMSSigErrDetDTC_raw32/1

== system ddm/DDM/DDM/VMC_DDM/CC Malfunction  ==
  task_time_s : Inport
  VDDM_BMSSigErrCFS_flg : Inport  Port=2
  VDDM_FrMCUSigErrCFS_flg : Inport  Port=3
  VDDM_RrMCUSigErrCFS_flg : Inport  Port=4
  VDDM_CCUSigErrCFS_flg : Inport  Port=5
  VDDM_ZoneSCPNoComCFS_flg : Inport  Port=6
  VDDM_MCUR1NoComCFS_flg : Inport  Port=7
  VDDM_MCUR1RCErrCFS_flg : Inport  Port=8
  VDDM_MCUR1CSErrCFS_flg : Inport  Port=9
  VDDM_MCUF1NoComCFS_flg : Inport  Port=10
  VDDM_MCUF1RCErrCFS_flg : Inport  Port=11
  VDDM_MCUF1CSErrCFS_flg : Inport  Port=12
  VDDM_ESC7NoComCFS_flg : Inport  Port=13
  VDDM_ESC7RCErrCFS_flg : Inport  Port=14
  VDDM_ESC7CSErrCFS_flg : Inport  Port=15
  VDDM_ESC1NoComCFS_flg : Inport  Port=16
  VDDM_ESC1RCErrCFS_flg : Inport  Port=17
  VDDM_ESC1CSErrCFS_flg : Inport  Port=18
  VDDM_ESC5NoComCFS_flg : Inport  Port=19
  VDDM_ESC5RCErrCFS_flg : Inport  Port=20
  VDDM_ESC5CSErrCFS_flg : Inport  Port=21
  No_CAN1_BUS_OFF : Inport  Port=22
  No_CAN3_BUS_OFF : Inport  Port=23
  No_CAN4_BUS_OFF : Inport  Port=24
  VPMM_PowerSta_enum : Inport  Port=25
  VINP_ZoneSpdCtrlMode_enum : Inport  Port=26
  DTC_clear_request : Inport  Port=27
  "CC Malfunction " : Subsystem
  From5 : From  Commented=on  GotoTag=VDDM_CCMalfuncDFS_flg
  Terminator : Terminator
  VDDM_CCMalfuncCFS_flg : Outport
  VDDM_CCMalfuncDetDTC_raw32 : Outport  Port=2
  wires:
  VDDM_BMSSigErrCFS_flg/1 -> [VDDM_BMSSigErrCFS_flg]
  [VDDM_CCMalfuncCFS_flg] -> VDDM_CCMalfuncCFS_flg/1
  From5/1 -> Terminator/1
  "CC Malfunction "/1(VDDM_CCMalfuncCFS_flg) -> [VDDM_CCMalfuncCFS_flg]
  VPMM_PowerSta_enum/1 -> [VPMM_PowerSta_enum]
  No_CAN1_BUS_OFF/1 -> [No_CAN1_BUS_OFF]
  VINP_ZoneSpdCtrlMode_enum/1 -> [VINP_ZoneSpdCtrlMode_enum]
  task_time_s/1 -> [task_time_s]  "task_time_s"
  VDDM_FrMCUSigErrCFS_flg/1 -> [VDDM_FrMCUSigErrCFS_flg]
  VDDM_RrMCUSigErrCFS_flg/1 -> [VDDM_RrMCUSigErrCFS_flg]
  VDDM_CCUSigErrCFS_flg/1 -> [VDDM_CCUSigErrCFS_flg]
  VDDM_ZoneSCPNoComCFS_flg/1 -> [VDDM_ZoneSCPNoComCFS_flg]
  VDDM_ESC7CSErrCFS_flg/1 -> [VDDM_ESC7CSErrCFS_flg]
  VDDM_ESC7RCErrCFS_flg/1 -> [VDDM_ESC7RCErrCFS_flg]
  VDDM_ESC7NoComCFS_flg/1 -> [VDDM_ESC7NoComCFS_flg]
  VDDM_ESC1NoComCFS_flg/1 -> [VDDM_ESC1NoComCFS_flg]
  VDDM_ESC1RCErrCFS_flg/1 -> [VDDM_ESC1RCErrCFS_flg]
  VDDM_ESC1CSErrCFS_flg/1 -> [VDDM_ESC1CSErrCFS_flg]
  VDDM_MCUF1CSErrCFS_flg/1 -> [VDDM_MCUF1CSErrCFS_flg]
  VDDM_MCUF1RCErrCFS_flg/1 -> [VDDM_MCUF1RCErrCFS_flg]
  VDDM_MCUF1NoComCFS_flg/1 -> [VDDM_MCUF1NoComCFS_flg]
  VDDM_MCUR1NoComCFS_flg/1 -> [VDDM_MCUR1NoComCFS_flg]
  VDDM_MCUR1RCErrCFS_flg/1 -> [VDDM_MCUR1RCErrCFS_flg]
  VDDM_MCUR1CSErrCFS_flg/1 -> [VDDM_MCUR1CSErrCFS_flg]
  VDDM_ESC5CSErrCFS_flg/1 -> [VDDM_ESC5CSErrCFS_flg]
  VDDM_ESC5RCErrCFS_flg/1 -> [VDDM_ESC5RCErrCFS_flg]
  VDDM_ESC5NoComCFS_flg/1 -> [VDDM_ESC5NoComCFS_flg]
  No_CAN3_BUS_OFF/1 -> [No_CAN3_BUS_OFF]
  No_CAN4_BUS_OFF/1 -> [No_CAN4_BUS_OFF]
  DTC_clear_request/1 -> [DTC_clear_request]
  [task_time_s] -> "CC Malfunction "/1(task_time_s)
  [VDDM_BMSSigErrCFS_flg] -> "CC Malfunction "/2(VDDM_BMSSigErrCFS_flg)
  [VDDM_FrMCUSigErrCFS_flg] -> "CC Malfunction "/3(VDDM_FrMCUSigErrCFS_flg)
  [VDDM_RrMCUSigErrCFS_flg] -> "CC Malfunction "/4(VDDM_RrMCUSigErrCFS_flg)
  [VDDM_CCUSigErrCFS_flg] -> "CC Malfunction "/5(VDDM_CCUSigErrCFS_flg)
  [VDDM_ZoneSCPNoComCFS_flg] -> "CC Malfunction "/6(VDDM_ZoneSCPNoComCFS_flg)
  [VDDM_MCUR1NoComCFS_flg] -> "CC Malfunction "/7(VDDM_MCUR1NoComCFS_flg)
  [VDDM_MCUR1RCErrCFS_flg] -> "CC Malfunction "/8(VDDM_MCUR1RCErrCFS_flg)
  [VDDM_MCUR1CSErrCFS_flg] -> "CC Malfunction "/9(VDDM_MCUR1CSErrCFS_flg)
  [VDDM_MCUF1NoComCFS_flg] -> "CC Malfunction "/10(VDDM_MCUF1NoComCFS_flg)
  [VDDM_MCUF1RCErrCFS_flg] -> "CC Malfunction "/11(VDDM_MCUF1RCErrCFS_flg)
  [VDDM_MCUF1CSErrCFS_flg] -> "CC Malfunction "/12(VDDM_MCUF1CSErrCFS_flg)
  [VDDM_ESC7NoComCFS_flg] -> "CC Malfunction "/13(VDDM_ESC7NoComCFS_flg)
  [VDDM_ESC7RCErrCFS_flg] -> "CC Malfunction "/14(VDDM_ESC7RCErrCFS_flg)
  [VDDM_ESC7CSErrCFS_flg] -> "CC Malfunction "/15(VDDM_ESC7CSErrCFS_flg)
  [VDDM_ESC1NoComCFS_flg] -> "CC Malfunction "/16(VDDM_ESC1NoComCFS_flg)
  [VDDM_ESC1RCErrCFS_flg] -> "CC Malfunction "/17(VDDM_ESC1RCErrCFS_flg)
  [VDDM_ESC1CSErrCFS_flg] -> "CC Malfunction "/18(VDDM_ESC1CSErrCFS_flg)
  [VDDM_ESC5NoComCFS_flg] -> "CC Malfunction "/19(VDDM_ESC5NoComCFS_flg)
  [VDDM_ESC5RCErrCFS_flg] -> "CC Malfunction "/20(VDDM_ESC5RCErrCFS_flg)
  [VDDM_ESC5CSErrCFS_flg] -> "CC Malfunction "/21(VDDM_ESC5CSErrCFS_flg)
  [No_CAN1_BUS_OFF] -> "CC Malfunction "/22(No_CAN1_BUS_OFF)
  [No_CAN3_BUS_OFF] -> "CC Malfunction "/23(No_CAN3_BUS_OFF)
  [No_CAN4_BUS_OFF] -> "CC Malfunction "/24(No_CAN4_BUS_OFF)
  [VPMM_PowerSta_enum] -> "CC Malfunction "/25(VPMM_PowerSta_enum)
  [VINP_ZoneSpdCtrlMode_enum] -> "CC Malfunction "/26(VINP_ZoneSpdCtrlMode_enum)
  [DTC_clear_request] -> "CC Malfunction "/27(DTC_clear_request)
  "CC Malfunction "/2(VDDM_CCMalfuncDetDTC_raw32) -> [VDDM_CCMalfuncDetDTC_raw32]
  [VDDM_CCMalfuncDetDTC_raw32] -> VDDM_CCMalfuncDetDTC_raw32/1

== system ddm/DDM/DDM/VMC_DDM/CCU Signal Error ==
  task_time_s : Inport
  VDDM_C3CCU2LCCFS_flg : Inport  Port=2
  VDDM_C3CCU2RCCFS_flg : Inport  Port=3
  VDDM_C3CCU2CSCFS_flg : Inport  Port=4
  No_CAN_BUS_OFF : Inport  Port=5
  VPMM_PowerSta_enum : Inport  Port=6
  VINP_DCDCFaultSta_enum : Inport  Port=7
  DTC_clear_request : Inport  Port=8
  "CCU Signal Error " : Subsystem
  From5 : From  Commented=on  GotoTag=VDDM_CCUSigErrDFS_flg
  Terminator : Terminator
  VDDM_CCUSigErrCFS_flg : Outport
  VDDM_CCUSigErrDetDTC_raw32 : Outport  Port=2
  wires:
  VDDM_C3CCU2CSCFS_flg/1 -> [VDDM_C3CCU2CSCFS_flg]
  VDDM_C3CCU2RCCFS_flg/1 -> [VDDM_C3CCU2RCCFS_flg]
  [VDDM_CCUSigErrCFS_flg] -> VDDM_CCUSigErrCFS_flg/1
  From5/1 -> Terminator/1
  "CCU Signal Error "/1(VDDM_CCUSigErrCFS_flg) -> [VDDM_CCUSigErrCFS_flg]
  DTC_clear_request/1 -> [DTC_clear_request]
  VPMM_PowerSta_enum/1 -> [VPMM_PowerSta_enum]
  No_CAN_BUS_OFF/1 -> [No_CAN_BUS_OFF]
  VDDM_C3CCU2LCCFS_flg/1 -> [VDDM_C3CCU2LCCFS_flg]
  VINP_DCDCFaultSta_enum/1 -> [VINP_DCDCFaultSta_enum]
  [VDDM_C3CCU2LCCFS_flg] -> "CCU Signal Error "/2(VDDM_C3CCU2LCCFS_flg)
  [VDDM_C3CCU2RCCFS_flg] -> "CCU Signal Error "/3(VDDM_C3CCU2RCCFS_flg)
  [VDDM_C3CCU2CSCFS_flg] -> "CCU Signal Error "/4(VDDM_C3CCU2CSCFS_flg)
  [No_CAN_BUS_OFF] -> "CCU Signal Error "/5(No_CAN_BUS_OFF)
  [VPMM_PowerSta_enum] -> "CCU Signal Error "/6(VPMM_PowerSta_enum)
  [VINP_DCDCFaultSta_enum] -> "CCU Signal Error "/7(VINP_DCDCFaultSta_enum)
  [DTC_clear_request] -> "CCU Signal Error "/8(DTC_clear_request)
  task_time_s/1 -> [task_time_s]  "task_time_s"
  [task_time_s] -> "CCU Signal Error "/1(task_time_s)
  "CCU Signal Error "/2(VDDM_CCUSigErrDetDTC_raw32) -> [VDDM_CCUSigErrDetDTC_raw32]
  [VDDM_CCUSigErrDetDTC_raw32] -> VDDM_CCUSigErrDetDTC_raw32/1

== system ddm/DDM/DDM/VMC_DDM/FCM2 ==
  task_time_s : Inport
  VDDM_FCM2NoCom_flg : Inport  Port=2
  VDDM_FCM2RCErr_flg : Inport  Port=3
  VDDM_FCM2CSErr_flg : Inport  Port=4
  No_CAN_BUS_OFF : Inport  Port=5
  VPMM_PowerSta_enum : Inport  Port=6
  VINP_ADASACCSta_enum : Inport  Port=7
  DTC_clear_request : Inport  Port=8
  Constant18 : Constant  Commented=on  Value=TRUE
  Constant21 : Constant  Commented=on  Value=FALSE
  "FCM2 Checksum Error " : Subsystem
  FCM2 Lost Com : Subsystem
  "FCM2 Rolling Count Error " : Subsystem
  From15 : From  Commented=on  GotoTag=VDDM_FCM2NoComCFS_flg
  From16 : From  Commented=on  GotoTag=VDDM_FCM2RCErrCFS_flg
  From17 : From  Commented=on  GotoTag=VDDM_FCM2CSErrCFS_flg
  From30 : From  Commented=on  GotoTag=VDDM_VCUACCErr_flg
  Goto11 : Goto  Commented=on  GotoTag=VDDM_VCUACCErr_flg
  Logical Operator2 : Logic  Commented=on  Operator=OR  Inputs=3  AllPortsSameDT=off  OutDataTypeStr=boolean
  Switch : Switch  Commented=on  Criteria=u2 ~= 0
  Terminator : Terminator
  VDDM_FCM2NoComDFS_flg : Outport
  VDDM_FCM2NoComCFS_flg : Outport  Port=2
  VDDM_FCM2RCErrDFS_flg : Outport  Port=3
  VDDM_FCM2RCErrCFS_flg : Outport  Port=4
  VDDM_FCM2CSErrDFS_flg : Outport  Port=5
  VDDM_FCM2CSErrCFS_flg : Outport  Port=6
  VDDM_FCM2NoComDTC_raw32 : Outport  Port=7
  VDDM_FCM2RCErrDTC_raw32 : Outport  Port=8
  VDDM_FCM2CSErrDTC_raw32 : Outport  Port=9
  wires:
  VDDM_FCM2NoCom_flg/1 -> [VDDM_FCM2NoCom_flg]
  [VDDM_FCM2NoCom_flg] -> FCM2 Lost Com/2(VDDM_FCM2NoCom_flg)
  No_CAN_BUS_OFF/1 -> [No_CAN_BUS_OFF]
  VPMM_PowerSta_enum/1 -> [VPMM_PowerSta_enum]
  VINP_ADASACCSta_enum/1 -> [VINP_ADASACCSta_enum]
  DTC_clear_request/1 -> [DTC_clear_request]
  [No_CAN_BUS_OFF] -> FCM2 Lost Com/3(No_CAN_BUS_OFF)
  [VPMM_PowerSta_enum] -> FCM2 Lost Com/4(VPMM_PowerSta_enum)
  [VINP_ADASACCSta_enum] -> FCM2 Lost Com/5(VINP_ADASACCSta_enum)
  [DTC_clear_request] -> FCM2 Lost Com/6(DTC_clear_request)
  FCM2 Lost Com/2(VDDM_FCM2NoComCFS_flg) -> [VDDM_FCM2NoComCFS_flg]
  FCM2 Lost Com/1(VDDM_FCM2NoComDFS_flg) -> [VDDM_FCM2NoComDFS_flg]
  [VDDM_FCM2NoComDFS_flg] -> VDDM_FCM2NoComDFS_flg/1
  [VDDM_FCM2NoComCFS_flg] -> "FCM2 Rolling Count Error "/4(VDDM_FCM2NoComCFS_flg)
  [VDDM_FCM2RCErr_flg] -> "FCM2 Rolling Count Error "/2(VDDM_FCM2RCErr_flg)
  [No_CAN_BUS_OFF] -> "FCM2 Rolling Count Error "/3(No_CAN_BUS_OFF)
  [VPMM_PowerSta_enum] -> "FCM2 Rolling Count Error "/5(VPMM_PowerSta_enum)
  [VINP_ADASACCSta_enum] -> "FCM2 Rolling Count Error "/6(VINP_ADASACCSta_enum)
  [DTC_clear_request] -> "FCM2 Rolling Count Error "/7(DTC_clear_request)
  "FCM2 Rolling Count Error "/1(VDDM_FCM2RCErrDFS_flg) -> [VDDM_FCM2RCErrDFS_flg]
  "FCM2 Rolling Count Error "/2(VDDM_FCM2RCErrCFS_flg) -> [VDDM_FCM2RCErrCFS_flg]
  [VDDM_FCM2NoComCFS_flg] -> VDDM_FCM2NoComCFS_flg/1
  [VDDM_FCM2CSErrDFS_flg] -> VDDM_FCM2CSErrDFS_flg/1
  [VDDM_FCM2CSErrCFS_flg] -> VDDM_FCM2CSErrCFS_flg/1
  [VDDM_FCM2RCErrCFS_flg] -> VDDM_FCM2RCErrCFS_flg/1
  [VDDM_FCM2RCErrDFS_flg] -> VDDM_FCM2RCErrDFS_flg/1
  Switch/1 -> Goto11/1
  From30/1 -> Terminator/1
  VDDM_FCM2RCErr_flg/1 -> [VDDM_FCM2RCErr_flg]
  VDDM_FCM2CSErr_flg/1 -> [VDDM_FCM2CSErr_flg]
  Constant18/1 -> Switch/1
  Constant21/1 -> Switch/3
  From15/1 -> Logical Operator2/1
  From16/1 -> Logical Operator2/2
  From17/1 -> Logical Operator2/3
  Logical Operator2/1 -> Switch/2
  [task_time_s] -> FCM2 Lost Com/1(task_time_s)
  task_time_s/1 -> [task_time_s]  "task_time_s"
  [task_time_s] -> "FCM2 Rolling Count Error "/1(task_time_s)
  [task_time_s] -> "FCM2 Checksum Error "/1(task_time_s)
  [DTC_clear_request] -> "FCM2 Checksum Error "/7(DTC_clear_request)
  [VINP_ADASACCSta_enum] -> "FCM2 Checksum Error "/6(VINP_ADASACCSta_enum)
  [VPMM_PowerSta_enum] -> "FCM2 Checksum Error "/5(VPMM_PowerSta_enum)
  [No_CAN_BUS_OFF] -> "FCM2 Checksum Error "/3(No_CAN_BUS_OFF)
  [VDDM_FCM2CSErr_flg] -> "FCM2 Checksum Error "/2(VDDM_FCM2CSErr_flg)
  [VDDM_FCM2NoComCFS_flg] -> "FCM2 Checksum Error "/4(VDDM_FCM2NoComCFS_flg)
  "FCM2 Checksum Error "/1(VDDM_FCM2CSErrDFS_flg) -> [VDDM_FCM2CSErrDFS_flg]
  "FCM2 Checksum Error "/2(VDDM_FCM2CSErrCFS_flg) -> [VDDM_FCM2CSErrCFS_flg]
  FCM2 Lost Com/3(VDDM_FCM2NoComDTC_raw32) -> [VDDM_FCM2NoComDTC_raw32]
  "FCM2 Rolling Count Error "/3(VDDM_FCM2RCErrDTC_raw32) -> [VDDM_FCM2RCErrDTC_raw32]
  "FCM2 Checksum Error "/3(VDDM_FCM2CSErrDTC_raw32) -> [VDDM_FCM2CSErrDTC_raw32]
  [VDDM_FCM2NoComDTC_raw32] -> VDDM_FCM2NoComDTC_raw32/1
  [VDDM_FCM2RCErrDTC_raw32] -> VDDM_FCM2RCErrDTC_raw32/1
  [VDDM_FCM2CSErrDTC_raw32] -> VDDM_FCM2CSErrDTC_raw32/1

== system ddm/DDM/DDM/VMC_DDM/FCM3 ==
  task_time_s : Inport
  VDDM_FCM3NoCom_flg : Inport  Port=2
  VDDM_FCM3RCErr_flg : Inport  Port=3
  VDDM_FCM3CSErr_flg : Inport  Port=4
  No_CAN_BUS_OFF : Inport  Port=5
  VPMM_PowerSta_enum : Inport  Port=6
  VINP_ADASACCSta_enum : Inport  Port=7
  VINP_ADASISASta_enum : Inport  Port=8
  DTC_clear_request : Inport  Port=9
  Constant18 : Constant  Commented=on  Value=TRUE
  Constant21 : Constant  Commented=on  Value=FALSE
  "FCM3 Checksum Error " : Subsystem
  FCM3 Lost Com : Subsystem
  "FCM3 Rolling Count Error " : Subsystem
  From15 : From  Commented=on  GotoTag=VDDM_FCM3NoComCFS_flg
  From16 : From  Commented=on  GotoTag=VDDM_FCM3RCErrCFS_flg
  From17 : From  Commented=on  GotoTag=VDDM_FCM3CSErrCFS_flg
  From23 : From  Commented=on  GotoTag=VDDM_VCUISAErr_flg
  Goto11 : Goto  Commented=on  GotoTag=VDDM_VCUISAErr_flg
  Logical Operator2 : Logic  Commented=on  Operator=OR  Inputs=3  AllPortsSameDT=off  OutDataTypeStr=boolean
  Switch : Switch  Commented=on  Criteria=u2 ~= 0
  Terminator : Terminator
  VDDM_FCM3NoComDFS_flg : Outport
  VDDM_FCM3NoComCFS_flg : Outport  Port=2
  VDDM_FCM3RCErrDFS_flg : Outport  Port=3
  VDDM_FCM3RCErrCFS_flg : Outport  Port=4
  VDDM_FCM3CSErrDFS_flg : Outport  Port=5
  VDDM_FCM3CSErrCFS_flg : Outport  Port=6
  VDDM_FCM3NoComDTC_raw32 : Outport  Port=7
  VDDM_FCM3RCErrDTC_raw32 : Outport  Port=8
  VDDM_FCM3CSErrDTC_raw32 : Outport  Port=9
  wires:
  VDDM_FCM3NoCom_flg/1 -> [VDDM_FCM3NoCom_flg]
  [VDDM_FCM3NoCom_flg] -> FCM3 Lost Com/2(VDDM_FCM3NoCom_flg)
  No_CAN_BUS_OFF/1 -> [No_CAN_BUS_OFF]
  VPMM_PowerSta_enum/1 -> [VPMM_PowerSta_enum]
  VINP_ADASACCSta_enum/1 -> [VINP_ADASACCSta_enum]
  DTC_clear_request/1 -> [DTC_clear_request]
  [No_CAN_BUS_OFF] -> FCM3 Lost Com/3(No_CAN_BUS_OFF)
  [VPMM_PowerSta_enum] -> FCM3 Lost Com/4(VPMM_PowerSta_enum)
  [VINP_ADASACCSta_enum] -> FCM3 Lost Com/5(VINP_ADASACCSta_enum)
  [DTC_clear_request] -> FCM3 Lost Com/7(DTC_clear_request)
  FCM3 Lost Com/2(VDDM_FCM3NoComCFS_flg) -> [VDDM_FCM3NoComCFS_flg]
  FCM3 Lost Com/1(VDDM_FCM3NoComDFS_flg) -> [VDDM_FCM3NoComDFS_flg]
  [VDDM_FCM3NoComDFS_flg] -> VDDM_FCM3NoComDFS_flg/1
  [VDDM_FCM3NoComCFS_flg] -> "FCM3 Rolling Count Error "/4(VDDM_FCM3NoComCFS_flg)
  [VDDM_FCM3RCErr_flg] -> "FCM3 Rolling Count Error "/2(VDDM_FCM3RCErr_flg)
  [No_CAN_BUS_OFF] -> "FCM3 Rolling Count Error "/3(No_CAN_BUS_OFF)
  [VPMM_PowerSta_enum] -> "FCM3 Rolling Count Error "/5(VPMM_PowerSta_enum)
  [VINP_ADASACCSta_enum] -> "FCM3 Rolling Count Error "/6(VINP_ADASACCSta_enum)
  [DTC_clear_request] -> "FCM3 Rolling Count Error "/8(DTC_clear_request)
  "FCM3 Rolling Count Error "/1(VDDM_FCM3RCErrDFS_flg) -> [VDDM_FCM3RCErrDFS_flg]
  "FCM3 Rolling Count Error "/2(VDDM_FCM3RCErrCFS_flg) -> [VDDM_FCM3RCErrCFS_flg]
  [VDDM_FCM3NoComCFS_flg] -> VDDM_FCM3NoComCFS_flg/1
  [VDDM_FCM3CSErrDFS_flg] -> VDDM_FCM3CSErrDFS_flg/1
  [VDDM_FCM3CSErrCFS_flg] -> VDDM_FCM3CSErrCFS_flg/1
  [VDDM_FCM3RCErrCFS_flg] -> VDDM_FCM3RCErrCFS_flg/1
  [VDDM_FCM3RCErrDFS_flg] -> VDDM_FCM3RCErrDFS_flg/1
  Switch/1 -> Goto11/1
  From23/1 -> Terminator/1
  VDDM_FCM3RCErr_flg/1 -> [VDDM_FCM3RCErr_flg]
  VDDM_FCM3CSErr_flg/1 -> [VDDM_FCM3CSErr_flg]
  Constant18/1 -> Switch/1
  Constant21/1 -> Switch/3
  From15/1 -> Logical Operator2/1
  From16/1 -> Logical Operator2/2
  From17/1 -> Logical Operator2/3
  Logical Operator2/1 -> Switch/2
  [task_time_s] -> FCM3 Lost Com/1(task_time_s)
  task_time_s/1 -> [task_time_s]  "task_time_s"
  [task_time_s] -> "FCM3 Rolling Count Error "/1(task_time_s)
  [task_time_s] -> "FCM3 Checksum Error "/1(task_time_s)
  [DTC_clear_request] -> "FCM3 Checksum Error "/8(DTC_clear_request)
  [VINP_ADASACCSta_enum] -> "FCM3 Checksum Error "/6(VINP_ADASACCSta_enum)
  [VPMM_PowerSta_enum] -> "FCM3 Checksum Error "/5(VPMM_PowerSta_enum)
  [No_CAN_BUS_OFF] -> "FCM3 Checksum Error "/3(No_CAN_BUS_OFF)
  [VDDM_FCM3CSErr_flg] -> "FCM3 Checksum Error "/2(VDDM_FCM3CSErr_flg)
  [VDDM_FCM3NoComCFS_flg] -> "FCM3 Checksum Error "/4(VDDM_FCM3NoComCFS_flg)
  "FCM3 Checksum Error "/1(VDDM_FCM3CSErrDFS_flg) -> [VDDM_FCM3CSErrDFS_flg]
  "FCM3 Checksum Error "/2(VDDM_FCM3CSErrCFS_flg) -> [VDDM_FCM3CSErrCFS_flg]
  [VINP_ADASISASta_enum] -> FCM3 Lost Com/6(VINP_ADASISASta_enum)
  VINP_ADASISASta_enum/1 -> [VINP_ADASISASta_enum]
  [VINP_ADASISASta_enum] -> "FCM3 Rolling Count Error "/7(VINP_ADASISASta_enum)
  [VINP_ADASISASta_enum] -> "FCM3 Checksum Error "/7(VINP_ADASISASta_enum)
  FCM3 Lost Com/3(VDDM_FCM3NoComDTC_raw32) -> [VDDM_FCM3NoComDTC_raw32]
  "FCM3 Rolling Count Error "/3(VDDM_FCM3RCErrDTC_raw32) -> [VDDM_FCM3RCErrDTC_raw32]
  "FCM3 Checksum Error "/3(VDDM_FCM3CSErrDTC_raw32) -> [VDDM_FCM3CSErrDTC_raw32]
  [VDDM_FCM3NoComDTC_raw32] -> VDDM_FCM3NoComDTC_raw32/1
  [VDDM_FCM3RCErrDTC_raw32] -> VDDM_FCM3RCErrDTC_raw32/1
  [VDDM_FCM3CSErrDTC_raw32] -> VDDM_FCM3CSErrDTC_raw32/1

== system ddm/DDM/DDM/VMC_DDM/FCM4 ==
  task_time_s : Inport
  VDDM_FCM4NoCom_flg : Inport  Port=2
  VDDM_FCM4CSErr_flg : Inport  Port=3
  No_CAN_BUS_OFF : Inport  Port=4
  VPMM_PowerSta_enum : Inport  Port=5
  VINP_ADASACCSta_enum : Inport  Port=6
  DTC_clear_request : Inport  Port=7
  Constant18 : Constant  Commented=on  Value=TRUE
  Constant21 : Constant  Commented=on  Value=FALSE
  "FCM4 Checksum Error " : Subsystem
  FCM4 Lost Com : Subsystem
  "FCM4 Rolling Count Error " : Subsystem  Commented=on
  From10 : From  Commented=on  GotoTag=VINP_ADASACCSta_enum
  From11 : From  Commented=on  GotoTag=DTC_clear_request
  From15 : From  Commented=on  GotoTag=VDDM_FCM4NoComCFS_flg
  From16 : From  Commented=on  GotoTag=VDDM_FCM4RCErrCFS_flg
  From17 : From  Commented=on  GotoTag=VDDM_FCM4CSErrCFS_flg
  From19 : From  Commented=on  GotoTag=task_time_s
  From21 : From  Commented=on  GotoTag=VDDM_FCM4RCErrCFS_flg
  From22 : From  Commented=on  GotoTag=VDDM_FCM4RCErrDFS_flg
  From30 : From  Commented=on  GotoTag=VDDM_VCUACCErr_flg
  From6 : From  Commented=on  GotoTag=VDDM_FCM4NoComCFS_flg
  From7 : From  Commented=on  GotoTag=VDDM_FCM4RCErr_flg
  From8 : From  Commented=on  GotoTag=No_CAN_BUS_OFF
  From9 : From  Commented=on  GotoTag=VPMM_PowerSta_enum
  Goto11 : Goto  Commented=on  GotoTag=VDDM_VCUACCErr_flg
  Goto12 : Goto  Commented=on  GotoTag=VDDM_FCM4RCErr_flg
  Goto7 : Goto  Commented=on  GotoTag=VDDM_FCM4RCErrCFS_flg
  Goto8 : Goto  Commented=on  GotoTag=VDDM_FCM4RCErrDFS_flg
  Ground : Ground
  Logical Operator2 : Logic  Commented=on  Operator=OR  Inputs=3  AllPortsSameDT=off  OutDataTypeStr=boolean
  Switch : Switch  Commented=on  Criteria=u2 ~= 0
  Terminator : Terminator
  Terminator1 : Terminator
  Terminator2 : Terminator
  VDDM_FCM4NoComDFS_flg : Outport
  VDDM_FCM4NoComCFS_flg : Outport  Port=2
  VDDM_FCM4CSErrDFS_flg : Outport  Port=3
  VDDM_FCM4CSErrCFS_flg : Outport  Port=4
  VDDM_FCM4NoComDTC_raw32 : Outport  Port=5
  VDDM_FCM4CSErrDTC_raw32 : Outport  Port=6
  wires:
  VDDM_FCM4NoCom_flg/1 -> [VDDM_FCM4NoCom_flg]
  [VDDM_FCM4NoCom_flg] -> FCM4 Lost Com/2(VDDM_FCM4NoCom_flg)
  No_CAN_BUS_OFF/1 -> [No_CAN_BUS_OFF]
  VPMM_PowerSta_enum/1 -> [VPMM_PowerSta_enum]
  VINP_ADASACCSta_enum/1 -> [VINP_ADASACCSta_enum]
  DTC_clear_request/1 -> [DTC_clear_request]
  [No_CAN_BUS_OFF] -> FCM4 Lost Com/3(No_CAN_BUS_OFF)
  [VPMM_PowerSta_enum] -> FCM4 Lost Com/4(VPMM_PowerSta_enum)
  [VINP_ADASACCSta_enum] -> FCM4 Lost Com/5(VINP_ADASACCSta_enum)
  [DTC_clear_request] -> FCM4 Lost Com/6(DTC_clear_request)
  FCM4 Lost Com/2(VDDM_FCM4NoComCFS_flg) -> [VDDM_FCM4NoComCFS_flg]
  FCM4 Lost Com/1(VDDM_FCM4NoComDFS_flg) -> [VDDM_FCM4NoComDFS_flg]
  [VDDM_FCM4NoComDFS_flg] -> VDDM_FCM4NoComDFS_flg/1
  From6/1 -> "FCM4 Rolling Count Error "/4(VDDM_FCM4NoComCFS_flg)
  From7/1 -> "FCM4 Rolling Count Error "/2(VDDM_FCM4RCErr_flg)
  From8/1 -> "FCM4 Rolling Count Error "/3(No_CAN_BUS_OFF)
  From9/1 -> "FCM4 Rolling Count Error "/5(VPMM_PowerSta_enum)
  From10/1 -> "FCM4 Rolling Count Error "/6(VINP_ADASACCSta_enum)
  From11/1 -> "FCM4 Rolling Count Error "/7(DTC_clear_request)
  "FCM4 Rolling Count Error "/1(VDDM_FCM4RCErrDFS_flg) -> Goto8/1
  "FCM4 Rolling Count Error "/2(VDDM_FCM4RCErrCFS_flg) -> Goto7/1
  [VDDM_FCM4NoComCFS_flg] -> VDDM_FCM4NoComCFS_flg/1
  [VDDM_FCM4CSErrDFS_flg] -> VDDM_FCM4CSErrDFS_flg/1
  [VDDM_FCM4CSErrCFS_flg] -> VDDM_FCM4CSErrCFS_flg/1
  From21/1 -> Terminator1/1
  From22/1 -> Terminator/1
  Switch/1 -> Goto11/1
  From30/1 -> Terminator2/1
  Ground/1 -> Goto12/1
  VDDM_FCM4CSErr_flg/1 -> [VDDM_FCM4CSErr_flg]
  Constant18/1 -> Switch/1
  Constant21/1 -> Switch/3
  From15/1 -> Logical Operator2/1
  From16/1 -> Logical Operator2/2
  From17/1 -> Logical Operator2/3
  Logical Operator2/1 -> Switch/2
  [task_time_s] -> FCM4 Lost Com/1(task_time_s)
  task_time_s/1 -> [task_time_s]  "task_time_s"
  From19/1 -> "FCM4 Rolling Count Error "/1(task_time_s)
  [task_time_s] -> "FCM4 Checksum Error "/1(task_time_s)
  [DTC_clear_request] -> "FCM4 Checksum Error "/7(DTC_clear_request)
  [VINP_ADASACCSta_enum] -> "FCM4 Checksum Error "/6(VINP_ADASACCSta_enum)
  [VPMM_PowerSta_enum] -> "FCM4 Checksum Error "/5(VPMM_PowerSta_enum)
  [No_CAN_BUS_OFF] -> "FCM4 Checksum Error "/3(No_CAN_BUS_OFF)
  [VDDM_FCM4CSErr_flg] -> "FCM4 Checksum Error "/2(VDDM_FCM4CSErr_flg)
  [VDDM_FCM4NoComCFS_flg] -> "FCM4 Checksum Error "/4(VDDM_FCM4NoComCFS_flg)
  "FCM4 Checksum Error "/1(VDDM_FCM4CSErrDFS_flg) -> [VDDM_FCM4CSErrDFS_flg]
  "FCM4 Checksum Error "/2(VDDM_FCM4CSErrCFS_flg) -> [VDDM_FCM4CSErrCFS_flg]
  FCM4 Lost Com/3(VDDM_FCM4NoComDTC_raw32) -> [VDDM_FCM4NoComDTC_raw32]
  "FCM4 Checksum Error "/3(VDDM_FCM4CSErrDTC_raw32) -> [VDDM_FCM4CSErrDTC_raw32]
  [VDDM_FCM4NoComDTC_raw32] -> VDDM_FCM4NoComDTC_raw32/1
  [VDDM_FCM4CSErrDTC_raw32] -> VDDM_FCM4CSErrDTC_raw32/1
